simulink model "parameter_sweep_M"  (R2020a)
settings: Solver=VariableStepAuto  StartTime=0.0  StopTime=2  RelTol=1e-3
values from neighbouring files (symbols this model uses):
  A_w = 1    [parameter_sweep_LRM_plotter.m]    (also in parameter_sweep_Mechanical_plotter.m)
  l_w = 1    [parameter_sweep_LRM_plotter.m]    (also in parameter_sweep_Mechanical_plotter.m)
  Nw = 4    [parameter_sweep_LRM_plotter.m]    (also in parameter_sweep_Mechanical_plotter.m = 300)
  R = 4.95    [parameter_sweep_LRM_plotter.m]    (also in parameter_sweep_LR_plotter.m = 7; parameter_sweep_M_plotter.m = 7; parameter_sweep_Mechanical_plotter.m = 5)
  R_Int = 0.55    [parameter_sweep_LRM_plotter.m]    (also in parameter_sweep_Mechanical_plotter.m = 0.33)
  Rel = Nw^2/ (0.004)    (= 4000)    [parameter_sweep_LRM_plotter.m]    (also in parameter_sweep_M_plotter.m = 0 + ((i-1) * 10); parameter_sweep_Mechanical_plotter.m = 0)
  V_T = 33.5    [parameter_sweep_LRM_plotter.m]    (also in parameter_sweep_LR_plotter.m = 4 + ((i-1) * 1); parameter_sweep_M_plotter.m = 350; parameter_sweep_Mechanical_plotter.m)
undefined symbols (not defined in the file or in its folder): phi
libraries: fl_lib x12, nesl_utility x12, simulink x2
settings Model: Creator=insat  LastModifiedBy=gwb15193

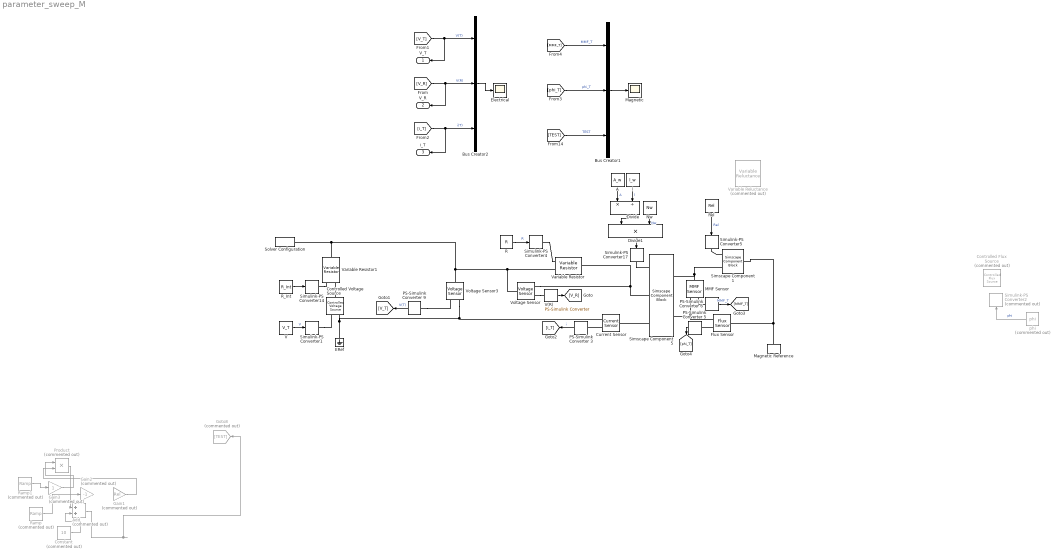
== system parameter_sweep_M ==
  A : Constant  Value=A_w
  Add : Sum  Commented=on
  Bus Creator1 : BusCreator  Inputs=3
  Bus Creator2 : BusCreator  Inputs=3
  Constant : Constant  Commented=on  Value=10
  Controlled Flux Source : fl_lib/Magnetic/Magnetic Sources/Controlled Flux Source  Commented=on
      settings: SourceProductBaseCode=SS  InternalSimscapePortConfiguration="{\"Bottom\":[],\"Left\":[{\"id\":\"N\",\"label\":\"\",\"type\":\"foundation.magnetic.magnetic\"}],\"Right\":[{\"id\":\"phiS\",\"label\":\"\",\"type\":\"input\"},{\"id\":\"S\",\"label\":\"\",\"type\":\"foundation.magnetic.magnetic\"}],\"Top\":[]}"
  Controlled Voltage Source : fl_lib/Electrical/Electrical Sources/Controlled Voltage Source
  Current Sensor : fl_lib/Electrical/Electrical Sensors/Current Sensor
  Divide : Product  Inputs=*/
  Divide1 : Product  Inputs=**
  ERef : fl_lib/Electrical/Electrical Elements/Electrical Reference
  Electrical : Scope
  Flux Sensor : fl_lib/Magnetic/Magnetic Sensors/Flux Sensor
      settings: SourceProductBaseCode=SS  InternalSimscapePortConfiguration="{\"Bottom\":[],\"Left\":[{\"id\":\"N\",\"label\":\"N\",\"type\":\"foundation.magnetic.magnetic\"}],\"Right\":[{\"id\":\"PHI\",\"label\":\"\",\"type\":\"output\"},{\"id\":\"S\",\"label\":\"S\",\"type\":\"foundation.magnetic.magnetic\"}],\"Top\":[]}"
  Gain1 : Gain  Commented=on  Gain=Rel
  Gain2 : Gain  Commented=on  Gain=-1
  Gain3 : Gain  Commented=on
  Goto8 : Goto  Commented=on  GotoTag=TEST
  MMF Sensor : fl_lib/Magnetic/Magnetic Sensors/MMF Sensor
      settings: SourceProductBaseCode=SS  InternalSimscapePortConfiguration="{\"Bottom\":[],\"Left\":[{\"id\":\"N\",\"label\":\"N\",\"type\":\"foundation.magnetic.magnetic\"}],\"Right\":[{\"id\":\"MMF\",\"label\":\"\",\"type\":\"output\"},{\"id\":\"S\",\"label\":\"S\",\"type\":\"foundation.magnetic.magnetic\"}],\"Top\":[]}"
  Magnetic : Scope
  Magnetic Reference : fl_lib/Magnetic/Magnetic Elements/Magnetic Reference
      settings: SourceProductBaseCode=SS  InternalSimscapePortConfiguration="{\"Bottom\":[],\"Left\":[{\"id\":\"M\",\"label\":\"\",\"type\":\"foundation.magnetic.magnetic\"}],\"Right\":[],\"Top\":[]}"
  Nw : Constant  Value=Nw
  PS-Simulink Converter 3 : nesl_utility/PS-Simulink Converter  PhysicalDomain=network_engine_domain  SubClassName=ps_output  LeftPortType=input  RightPortType=output  PseudoPeriodic=off  Frequencies=[]  Unit=A  AffineConversion=off
  PS-Simulink Converter 5 : nesl_utility/PS-Simulink Converter  PhysicalDomain=network_engine_domain  SubClassName=ps_output  LeftPortType=input  RightPortType=output  PseudoPeriodic=off  Frequencies=[]  Unit=Wb  AffineConversion=off
  PS-Simulink Converter 6 : nesl_utility/PS-Simulink Converter  PhysicalDomain=network_engine_domain  SubClassName=ps_output  LeftPortType=input  RightPortType=output  PseudoPeriodic=off  Frequencies=[]  Unit=A  AffineConversion=off
  PS-Simulink Converter 9 : nesl_utility/PS-Simulink Converter  PhysicalDomain=network_engine_domain  SubClassName=ps_output  LeftPortType=input  RightPortType=output  PseudoPeriodic=off  Frequencies=[]  Unit=V  AffineConversion=off
  Product : Product  Commented=on
  R : Constant  Value=R
  R_Int : Constant  Value=R_Int
  Ramp : simulink/Sources/Ramp  Commented=on  slope=1  start=0.01  InitialOutput=0
  Ramp1 : simulink/Sources/Ramp  Commented=on  slope=1  start=0.01  InitialOutput=0
  Rel : Constant  Value=Rel
  Simscape Component1 : SimscapeComponentBlock  SourceFile=fundamental_reluctance_mod  ComponentPath=fundamental_reluctance_mod  ComponentVariants="[\"fundamental_reluctance_mod\"]"  ComponentVariantNames="[\"fundamental_reluctance_mod\"]"  ClassName=fundamental_reluctance_mod  SchemaVersion=1  phi_specify=off  phi_priority=None  phi=0 Wb  phi_nominal_specify=off  phi_nominal_unit=Wb  phi_nominal_value=1  mmf_specify=off  mmf_priority=None  mmf=0 A  mmf_nominal_specify=off  mmf_nominal_unit=A  mmf_nominal_value=1
      settings: CopyFcn=simscape.engine.sli.internal.componentblockcallback(gcbh,'COPY')  PreCopyFcn=simscape.engine.sli.internal.componentblockcallback(gcbh,'PRECOPY')  PreDeleteFcn=simscape.engine.sli.internal.componentblockcallback(gcbh,'PREDELETE')  InternalSimscapePortConfiguration="{\"Bottom\":[],\"Left\":[{\"id\":\"N\",\"label\":\"N\",\"type\":\"foundation.magnetic.magnetic\"},{\"id\":\"R\",\"label\":\"Reluctance\",\"type\":\"input\"}],\"Right\":[{\"id\":\"S\",\"label\":\"S\",\"type\":\"foundation.magnetic.magnetic\"}],\"Top\":[]}"
      mask Type: Fundamental Reluctance
  Simscape Component5 : SimscapeComponentBlock  SourceFile=electromagenetic_converter_mod  ComponentPath=electromagenetic_converter_mod  ComponentVariants="[\"electromagenetic_converter_mod\"]"  ComponentVariantNames="[\"electromagenetic_converter_mod\"]"  ClassName=electromagenetic_converter_mod  SchemaVersion=1  i_specify=off  i_priority=None  i=0 A  i_nominal_specify=off  i_nominal_unit=A  i_nominal_value=1  v_specify=off  v_priority=None  v=0 V  v_nominal_specify=off  v_nominal_unit=V  v_nominal_value=1  mmf_specify=off  mmf_priority=None  mmf=0 A  mmf_nominal_specify=off  mmf_nominal_unit=A  mmf_nominal_value=1  phi_specify=off  phi_priority=High  phi=0 Wb  phi_nominal_specify=off  phi_nominal_unit=Wb  phi_nominal_value=1
      settings: CopyFcn=simscape.engine.sli.internal.componentblockcallback(gcbh,'COPY')  PreCopyFcn=simscape.engine.sli.internal.componentblockcallback(gcbh,'PRECOPY')  PreDeleteFcn=simscape.engine.sli.internal.componentblockcallback(gcbh,'PREDELETE')  InternalSimscapePortConfiguration="{\"Bottom\":[],\"Left\":[{\"id\":\"p\",\"label\":\"+\",\"type\":\"foundation.electrical.electrical\"},{\"id\":\"n\",\"label\":\"-\",\"type\":\"foundation.electrical.electrical\"},{\"id\":\"Nw\",\"label\":\"Number of winding turns\",\"type\":\"input\"}],\"Right\":[{\"id\":\"N\",\"label\":\"N\",\"type\":\"foundation.magnetic.magnetic\"},{\"id\":\"S\",\"label\":\"S\",\"type\":\"foundation.magnetic.magnetic\"}],\"Top\":[]}"
      mask Type: Electromagnetic Converter
  Simulink-PS Converter{1,4..5,14,17} (5 alike) : nesl_utility/Simulink-PS Converter  PhysicalDomain=network_engine_domain  SubClassName=ps_input  LeftPortType=input  RightPortType=output  PseudoPeriodic=off  Frequencies=[]  NoiseDistribution=none  NoiseParameters=[]  Unit=1  AffineConversion=off  FilteringAndDerivatives=zero  SimscapeFilterOrder=1  InputFilterTimeConstant=.001  UdotUserProvided=0
  Simulink-PS Converter2 : nesl_utility/Simulink-PS Converter  Commented=on  PhysicalDomain=network_engine_domain  SubClassName=ps_input  LeftPortType=input  RightPortType=output  PseudoPeriodic=off  Frequencies=[]  NoiseDistribution=none  NoiseParameters=[]  Unit=1  AffineConversion=off  FilteringAndDerivatives=zero  SimscapeFilterOrder=1  InputFilterTimeConstant=.001  UdotUserProvided=0
  Solver Configuration : nesl_utility/Solver Configuration  PhysicalDomain=network_engine_domain  SubClassName=solver  LeftPortType=input  RightPortType=generic  Tones=[]  Harmonics=[]  SimulateNoise=off  Profile=off  UseLocalSampling=off  EnableSwitchedLinearOptims=on  FrequencyDomain=off  UseCCode=off  RelTol=0.001  AbsTol=1e-06  MinStep=1e-09  ToWorkspace=off  RevertToSquareIcSolve=off  NumHomotopyIterations=100  PhasorMode=off  PhasorModeNumHarmonics=1  DoDC=off  ResidualTolerance=1e-9  UseLocalSolver=off  LocalSolverChoice=NE_BACKWARD_EULER_ADVANCER  LocalSolverSampleTime=.001  DoFixedCost=off  MaxNonlinIter=3  MaxModeIter=2  LinearAlgebra=auto  EquationFormulation=NE_TIME_EF  DelaysMemoryBudget=1024  AutomaticFiltering=on  FilteringTimeConstant=0.0001  PartitionStorageMethod=AS_NEEDED  PartitionMemoryBudget=1024  PartitionMethod=FAST
  V : Constant  Value=V_T
  V(R) : nesl_utility/PS-Simulink Converter  PhysicalDomain=network_engine_domain  SubClassName=ps_output  LeftPortType=input  RightPortType=output  PseudoPeriodic=off  Frequencies=[]  Unit=V  AffineConversion=off
  Variable Reluctance : fl_lib/Magnetic/Magnetic Elements/Variable Reluctance  Commented=on  Xmin=0.00000001 m  CSA=1 m^2  mur=1  phi_specify=off  phi_priority=None  phi=0 Wb  phi_nominal_specify=off  phi_nominal_unit=Wb  phi_nominal_value=1  mmf_specify=off  mmf_priority=None  mmf=0 A  mmf_nominal_specify=off  mmf_nominal_unit=A  mmf_nominal_value=1
      settings: SourceProductBaseCode=SS  InternalSimscapePortConfiguration="{\"Bottom\":[],\"Left\":[{\"id\":\"N\",\"label\":\"N\",\"type\":\"foundation.magnetic.magnetic\"},{\"id\":\"X\",\"label\":\"\",\"type\":\"input\"}],\"Right\":[{\"id\":\"S\",\"label\":\"S\",\"type\":\"foundation.magnetic.magnetic\"}],\"Top\":[]}"
  Variable Resistor : fl_lib/Electrical/Electrical Elements/Variable Resistor  Rmin=0 Ohm  i_specify=off  i_priority=None  i=0 A  i_nominal_specify=off  i_nominal_unit=A  i_nominal_value=1  v_specify=off  v_priority=None  v=0 V  v_nominal_specify=off  v_nominal_unit=V  v_nominal_value=1
  Variable Resistor1 : fl_lib/Electrical/Electrical Elements/Variable Resistor  Rmin=0 Ohm  i_specify=off  i_priority=None  i=0 A  i_nominal_specify=off  i_nominal_unit=A  i_nominal_value=1  v_specify=off  v_priority=None  v=0 V  v_nominal_specify=off  v_nominal_unit=V  v_nominal_value=1
  Voltage Sensor : fl_lib/Electrical/Electrical Sensors/Voltage Sensor
  Voltage Sensor3 : fl_lib/Electrical/Electrical Sensors/Voltage Sensor
  l : Constant  Value=l_w
  phi : Constant  Commented=on  Value=phi
  V_T : Outport  SignalName=V_T
  V_R : Outport  Port=2  SignalName=V_R
  i_T : Outport  Port=3  SignalName=i_T
  wires:
  V/1 -> Simulink-PS Converter1/1  "V"
  V(R)/1 -> [V_R]
  R/1 -> Simulink-PS Converter4/1  "R"
  PS-Simulink Converter 3/1 -> [i_T]  "i"
  PS-Simulink Converter 9/1 -> [V_T]  "V(T)"
  Bus Creator2/1 -> Electrical/1
  [i_T] -> i_T/1, Bus Creator2/3  "i(T)"
  [V_T] -> V_T/1, Bus Creator2/1  "V(T)"
  [V_R] -> V_R/1, Bus Creator2/2  "V(R)"
  PS-Simulink Converter 6/1 -> [MMF_T]  "MMF_T"
  [MMF_T] -> Bus Creator1/1  "MMF_T"
  [phi_T] -> Bus Creator1/2  "phi_T"
  Bus Creator1/1 -> Magnetic/1
  phi/1 -> Simulink-PS Converter2/1  "phi"
  [TEST] -> Bus Creator1/3  "TEST"
  R_Int/1 -> Simulink-PS Converter14/1
  Product/1 -> Add/1
  Add/1 -> Goto8/1
  Gain1/1 -> Product/2
  Ramp1/1 -> Gain3/1
  Gain3/1 -> Product/1
  Constant/1 -> Add/2
  Ramp/1 -> Gain2/1
  Rel/1 -> Simulink-PS Converter5/1  "Rel"
  Nw/1 -> Divide1/2  "Nw"
  Divide1/1 -> Simulink-PS Converter17/1
  Divide/1 -> Divide1/1
  A/1 -> Divide/1  "A"
  l/1 -> Divide/2  "l"
  PS-Simulink Converter 5/1 -> [phi_T]
  connections:
  ERef/LConn1 -- Current Sensor/RConn2 -- Voltage Sensor3/RConn2 -- Controlled Voltage Source/RConn2
  Voltage Sensor3/LConn1 -- Voltage Sensor/LConn1 -- Variable Resistor/LConn2 -- Variable Resistor1/RConn1 -- Solver Configuration/RConn1
  Voltage Sensor/RConn2 -- Variable Resistor/RConn1 -- Simscape Component5/LConn2
  Current Sensor/RConn1 -- PS-Simulink Converter 3/LConn1
  Voltage Sensor/RConn1 -- V(R)/LConn1
  Simulink-PS Converter1/RConn1 -- Controlled Voltage Source/RConn1
  PS-Simulink Converter 9/LConn1 -- Voltage Sensor3/RConn1
  Simulink-PS Converter4/RConn1 -- Variable Resistor/LConn1
  MMF Sensor/LConn1 -- Simscape Component1/LConn1 -- Simscape Component5/RConn2
  MMF Sensor/RConn2 -- Flux Sensor/RConn2 -- Simscape Component5/RConn1
  Simscape Component1/LConn2 -- Simulink-PS Converter5/RConn1
  PS-Simulink Converter 6/LConn1 -- MMF Sensor/RConn1
  Simscape Component5/LConn1 -- Current Sensor/LConn1
  Magnetic Reference/LConn1 -- Simscape Component1/RConn1 -- Flux Sensor/LConn1
  Variable Resistor1/LConn2 -- Controlled Voltage Source/LConn1
  Simulink-PS Converter14/RConn1 -- Variable Resistor1/LConn1
  Simulink-PS Converter17/RConn1 -- Simscape Component5/LConn3
  Flux Sensor/RConn1 -- PS-Simulink Converter 5/LConn1
